simulink model "Q10"  (R2021b)
settings: Solver=VariableStepAuto  StartTime=0.0  StopTime=10  RelTol=1e-3
undefined symbols (not defined in the file): C_new, D_new, deadbeat, G, H
settings Model: SimulationMode=accelerator  Creator=Siavash  LastModifiedBy=Siavash

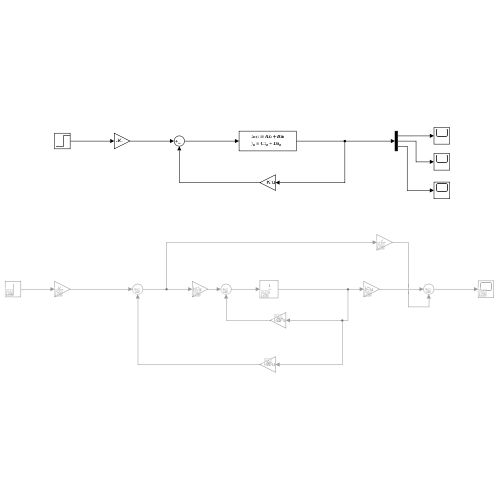
[thumbnail: Simulink's stored preview of the top-level diagram]
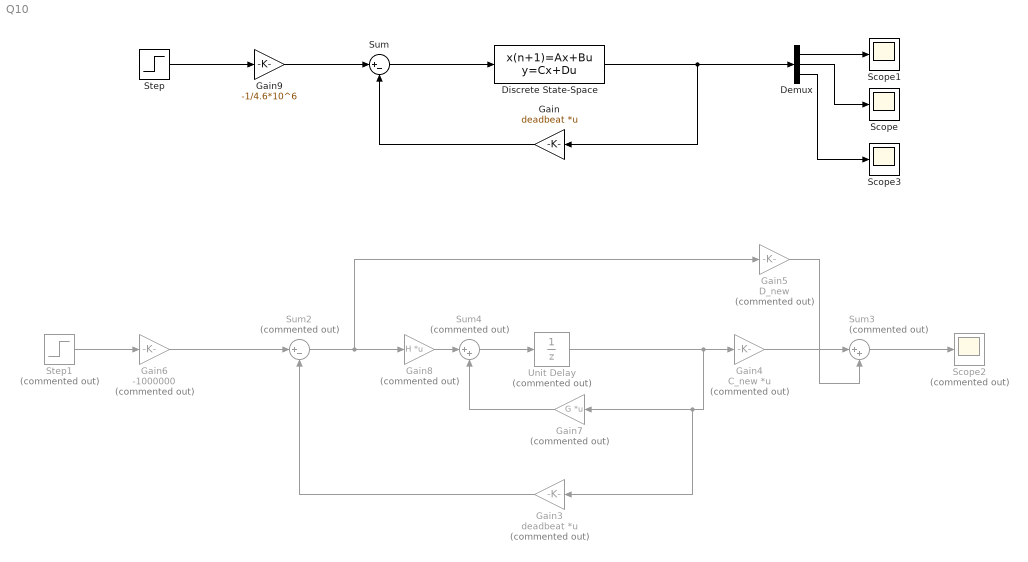
== system Q10 ==
  Demux : Demux  Outputs=3
  Discrete State-Space : DiscreteStateSpace  A=G  B=H  C=eye(3)  D=[0;0;0]
  Gain : Gain  Gain=deadbeat  Multiplication=Matrix(K*u)
  Gain3 : Gain  Commented=on  Gain=deadbeat  Multiplication=Matrix(K*u)
  Gain4 : Gain  Commented=on  Gain=C_new  Multiplication=Matrix(K*u)
  Gain5 : Gain  Commented=on  Gain=D_new
  Gain6 : Gain  Commented=on  Gain=-1000000
  Gain7 : Gain  Commented=on  Gain=G  Multiplication=Matrix(K*u)
  Gain8 : Gain  Commented=on  Gain=H  Multiplication=Matrix(K*u)
  Gain9 : Gain  Gain=-1/4.6*10^6
  Scope : Scope
  Scope1 : Scope
  Scope2 : Scope  Commented=on
  Scope3 : Scope
  Step : Step  SampleTime=0
  Step1 : Step  Commented=on  Time=0  SampleTime=0
  Sum : Sum  Inputs=|+-
  Sum2 : Sum  Commented=on  Inputs=|+-
  Sum3 : Sum  Commented=on  Inputs=|++
  Sum4 : Sum  Commented=on  Inputs=|++
  Unit Delay : UnitDelay  Commented=on  HasFrameUpgradeWarning=on
  wires:
  Discrete State-Space/1 -> Demux/1, Gain/1
  Gain/1 -> Sum/2
  Sum/1 -> Discrete State-Space/1
  Demux/1 -> Scope1/1
  Gain3/1 -> Sum2/2
  Sum3/1 -> Scope2/1
  Gain5/1 -> Sum3/2
  Gain4/1 -> Sum3/1
  Sum2/1 -> Gain5/1, Gain8/1
  Unit Delay/1 -> Gain4/1, Gain3/1, Gain7/1
  Gain7/1 -> Sum4/2
  Sum4/1 -> Unit Delay/1
  Gain8/1 -> Sum4/1
  Step1/1 -> Gain6/1
  Gain6/1 -> Sum2/1
  Step/1 -> Gain9/1
  Gain9/1 -> Sum/1
  Demux/2 -> Scope/1
  Demux/3 -> Scope3/1
